simulink model "Active"  (R2019a)
settings: Solver=ode113  StartTime=0.0  StopTime=20.0  RelTol=1e-3
values from neighbouring files (symbols this model uses):
  b1 = 600    [code.m]
  b2 = 800    [code.m]
  k1 = 18000    [code.m]
  k2 = 1950000    [code.m]
  m1 = 350    [code.m]
  m2 = 40    [code.m]
libraries: simulink x1
settings Model: Creator=DEVASHISH  LastModifiedBy=DEVASHISH
settings SolverCC: MaxConsecutiveMinStep=10

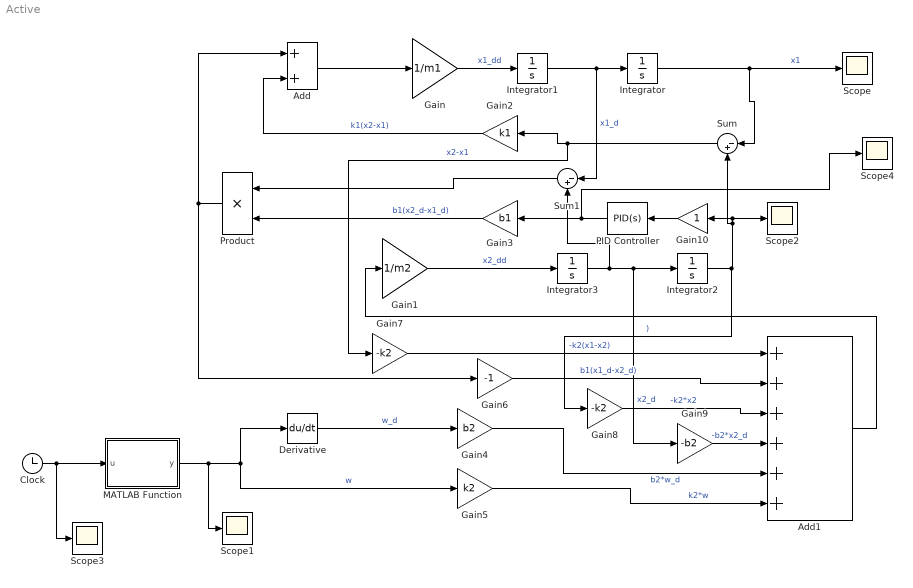
== system Active ==
  Add : Sum
  Add1 : Sum  Inputs=++++++
  Clock : Clock
  Derivative : Derivative
  Gain : Gain  Gain=1/m1
  Gain1 : Gain  Gain=1/m2
  Gain10 : Gain
  Gain2 : Gain  Gain=k1
  Gain3 : Gain  Gain=b1
  Gain4 : Gain  Gain=b2
  Gain5 : Gain  Gain=k2
  Gain6 : Gain  Gain=-1
  Gain7 : Gain  Gain=-k2
  Gain8 : Gain  Gain=-k2
  Gain9 : Gain  Gain=-b2
  Integrator{,1..3} (4 alike) : Integrator
  MATLAB Function : MATLAB Function  TreatAsAtomicUnit=on
  PID Controller : simulink/Continuous/PID Controller  Controller=PID  Form=Parallel  TimeDomain=Continuous-time  SampleTime=-1  IntegratorMethod=Forward Euler  FilterMethod=Forward Euler  ControllerParametersSource=internal  P=50  I=65  D=70  UseFilter=on  N=1  TunerSelectOption=Transfer Function Based (PID Tuner App)  InitialConditionSource=internal  InitialConditionForIntegrator=0  InitialConditionForFilter=0  DifferentiatorICPrevScaledInput=0  ExternalReset=none  TrackingMode=off  Kt=1  LimitOutput=on  UpperSaturationLimit=12  LowerSaturationLimit=0.1  LinearizeAsGain=on  AntiWindupMode=clamping  Kb=5  POutMin=[]  POutMax=[]  IOutMin=[]  IOutMax=[]  DOutMin=[]  DOutMax=[]  NOutMin=[]  NOutMax=[]  SumOutMin=[]  SumOutMax=[]  SaturationOutMin=[]  SaturationOutMax=[]  PParamMin=[]  PParamMax=[]  IParamMin=[]  IParamMax=[]  DParamMin=[]  DParamMax=[]  NParamMin=[]  NParamMax=[]  KbParamMin=[]  KbParamMax=[]  KtParamMin=[]  KtParamMax=[]  KbOutMin=[]  KbOutMax=[]  KtOutMin=[]  KtOutMax=[]  IntegratorOutMin=[]  IntegratorOutMax=[]  FilterOutMin=[]  FilterOutMax=[]  SumI1OutMin=[]  SumI1OutMax=[]  SumI2OutMin=[]  SumI2OutMax=[]  SumI3OutMin=[]  SumI3OutMax=[]  SumI4OutMin=[]  SumI4OutMax=[]  SumDOutMin=[]  SumDOutMax=[]  DifferentiatorOutMin=[]  DifferentiatorOutMax=[]  FilterDiffOutCoefMin=[]  FilterDiffOutCoefMax=[]  ReciprocalOutMin=[]  ReciprocalOutMax=[]  SumDenOutMin=[]  SumDenOutMax=[]  SumNumOutMin=[]  SumNumOutMax=[]  DivideOutMin=[]  DivideOutMax=[]  IntegratorContinuousStateAttributes=''  IntegratorStateMustResolveToSignalObject=off  IntegratorRTWStateStorageClass=Auto  FilterContinuousStateAttributes=''  FilterStateMustResolveToSignalObject=off  FilterRTWStateStorageClass=Auto  ParallelPVariant=InternalParameters  IdealPVariant=Disabled  IVariant=InternalParameters  DVariant=InternalParameters  IntegratorVariant=Continuous  SatVariant=Enabled  AWVariant=ContClampingParallel  PCopyVariant=Disabled  TRVariant=Disabled  FdbkBlocksVariant=Forward  IdealPFdbkVariant=Disabled  SatFdbkVariant=Disabled  DerivativeFilterVariant=ContFilter  NVariant=InternalParameters  NCopyVariant=Disabled  FilterICVariant=InternalICsFilter  IntegratorICVariant=InternalICs  ExternalResetVariant=Disabled  TRSumVariant=Passthrough  SumFdbkVariant=Disabled  SumVariant=Sum_PID
  Product : Product
  Scope{,1..4} (5 alike) : Scope
  Sum : Sum  Inputs=|-+
  Sum1 : Sum  Inputs=|-+
  wires:
  Gain4/1 -> Add1/5  "b2*w_d"
  Gain5/1 -> Add1/6  "k2*w"
  MATLAB Function/1(y) -> Scope1/1, Derivative/1, Gain5/1  "w"
  Gain6/1 -> Add1/2  "b1(x1_d-x2_d)"
  Gain7/1 -> Add1/1  "-k2(x1-x2)"
  Derivative/1 -> Gain4/1  "w_d"
  Gain9/1 -> Add1/4  "-b2*x2_d"
  Add/1 -> Gain/1
  Integrator1/1 -> Sum1/1, Integrator/1  "x1_d"
  Add1/1 -> Gain1/1
  Integrator/1 -> Sum/1, Scope/1  "x1"
  Gain1/1 -> Integrator3/1  "x2_dd"
  Sum/1 -> Gain7/1, Gain2/1  "x2-x1"
  Integrator3/1 -> Sum1/2, Gain9/1, Integrator2/1  "x2_d"
  Gain2/1 -> Add/2  "k1(x2-x1)"
  Gain8/1 -> Add1/3  "-k2*x2"
  Gain/1 -> Integrator1/1  "x1_dd"
  PID Controller/1 -> Scope4/1, Gain3/1
  Gain3/1 -> Product/2  "b1(x2_d-x1_d)"
  Sum1/1 -> Product/1
  Product/1 -> Add/1, Gain6/1
  Clock/1 -> Scope3/1, MATLAB Function/1(u)
  Integrator2/1 -> Gain10/1, Scope2/1, Sum/2, Gain8/1  ")"
  Gain10/1 -> PID Controller/1

== matlab function Active/MATLAB Function ==
  data: u input; y output
function y = fcn(u)
%if u>2
%y=1;
%if   u>5 && u<10
%y=-0.1*(5*(u-5)-(u-10))*sin(0.2*pi*u);
if u<8
    y=sin(0.25*pi*u);
else
y=0;
end
end
